simulink model "simple_kafka_consumer_producer_example"  (R2018a)
settings: Solver=FixedStepAuto  StartTime=0.0  StopTime=inf  RelTol=1e-3
libraries: simulink x5, sl_kafka_lib x4
settings Model: EnablePacing=on  Creator=asolland  LastModifiedBy=asolland
settings OptimizationCC: DefaultParameterBehavior=Inlined  EnhancedBackFolding=on  PassReuseOutputArgsAs=Individual arguments  OptimizeBlockOrder=speed  DifferentSizesBufferReuse=on  OptimizationCustomize=off
settings DebuggingCC: ParameterTunabilityLossMsg=error
settings HardwareCC: ProdBitPerLong=64  ProdLongLongMode=on  ProdHWDeviceType=Intel->x86-64 (Linux 64)
settings SFSimCC: SimUseLocalCustomCode=on  MATLABDynamicMemAlloc=off
settings RTWCC: Description=Kafka Target  SystemTargetFile=kafkatarget.tlc  TemplateMakefile=ert_default_tmf  GenerateReport=on  RetainRTWFile=on  RTWUseLocalCustomCode=on  IncludeHyperlinkInReport=on  LaunchReport=on  GenerateTraceInfo=on  GenerateTraceReport=on  GenerateTraceReportSl=on  GenerateTraceReportSf=on  GenerateTraceReportEml=on
settings CodeAppCC: ForceParamTrailComments=on  IgnoreCustomStorageClasses=off  OperatorAnnotations=on  SimulinkDataObjDesc=on  SFDataObjDesc=on  InsertBlockDesc=on
settings STFCustomTargetCC: TargetLangStandard=C99 (ISO)  MultiwordLength=256  GenerateSampleERTMain=on  CombineOutputUpdateFcns=on  ERTCustomFileBanners=on  SupportContinuousTime=off  SupportNonInlinedSFcns=off  RemoveResetFunc=on  MATLABClassNameForMDSCustomization=Simulink.SoftwareTarget.ERTCustomization  GRTInterface=off  UseToolchainInfoCompliant=on  SystemTargetFile=kafkatarget.tlc
settings ERTTargetCC: TargetLangStandard=C99 (ISO)  GenerateSampleERTMain=on  ParMdlRefBuildCompliant=off  CompOptLevelCompliant=off  ConcurrentExecutionCompliant=off  ModelStepFunctionPrototypeControlCompliant=off  CPPClassGenCompliant=off  InlinedParameterPlacement=NonHierarchical  ERTCustomFileTemplate=kafkatarget_process.tlc

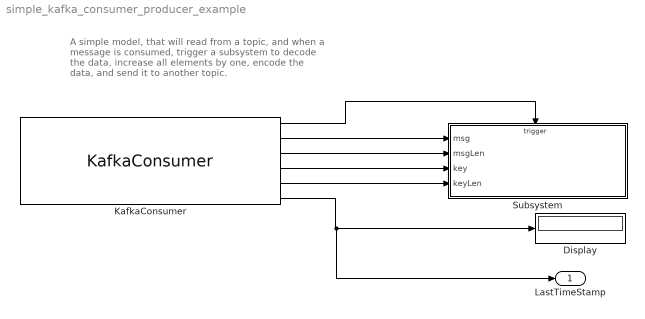
== system simple_kafka_consumer_producer_example ==
  note: A simple model, that will read from a topic, and
      | when a message is consumed, trigger a subsystem
      | to decode the data, increase all elements by one,
      | encode the data, and send it to another topic.
  Display : Display
  KafkaConsumer : sl_kafka_lib/KafkaConsumer  sfpBrokers='localhost:9092'  sfpTopic='sltopic'  sfpGroup='abc'  sfpMsgLen=200  sfpKeyLen=32  sfpOutputTimestamp=on  sfpTS=1e-3  sfpConf=|  sfpTopicConf=compression.level=-1
      | client.id=sl_kafka_consumer
      | message.copy.max.bytes=65535
      settings: SourceProductName=Kafka Library
  Subsystem : Subsystem
  LastTimeStamp : Outport  VectorParamsAs1DForOutWhenUnconnected=off
  wires:
  KafkaConsumer/2 -> Subsystem/1(msg)
  KafkaConsumer/3 -> Subsystem/2(msgLen)
  KafkaConsumer/4 -> Subsystem/3(key)
  KafkaConsumer/5 -> Subsystem/4(keyLen)
  KafkaConsumer/1 -> Subsystem/Trigger
  KafkaConsumer/6 -> LastTimeStamp/1, Display/1

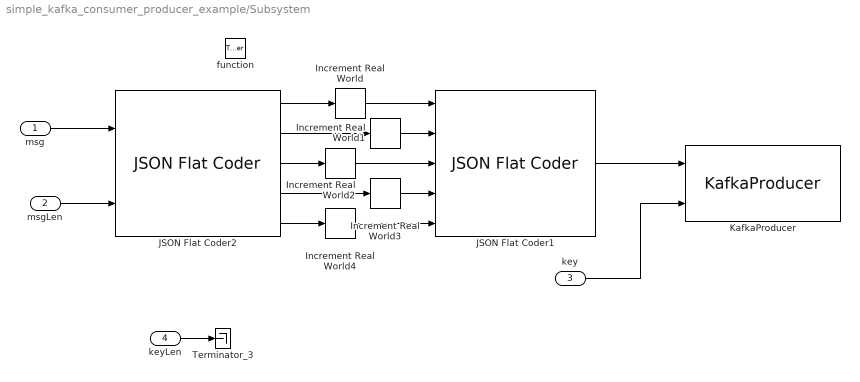
== system simple_kafka_consumer_producer_example/Subsystem ==
  msg : Inport
  msgLen : Inport  Port=2
  key : Inport  Port=3
  keyLen : Inport  Port=4
  function : TriggerPort  TriggerType=function-call  VariantControl=Variant
  Increment Real World{,1..4} (5 alike) : simulink/Additional Math & Discrete/Additional Math: Increment - Decrement/Increment Real World
      settings: SourceProductName=Simulink  SourceProductBaseCode=SL
  JSON Flat Coder1 : sl_kafka_lib/JSON Flat Coder  sfpDirection=Encode  sfpLength=200  sfpFields={'TS', 'M', 'Flow', 'Pressure', 'Current'}  sfpOutLength=off  sfpInLength=on
      settings: SourceProductName=Kafka Library
  JSON Flat Coder2 : sl_kafka_lib/JSON Flat Coder  sfpDirection=Decode  sfpLength=200  sfpFields={'TS', 'M', 'Flow', 'Pressure', 'Current'}  sfpOutLength=on  sfpInLength=on
      settings: SourceProductName=Kafka Library
  KafkaProducer : sl_kafka_lib/KafkaProducer  sfpBrokers='localhost:9092'  sfpTopic='sltopic2'  sfpKeyAsInput=on  sfpKeyAsInputLen=32  sfpKey='key1'  sfpMsgLen=200  sfpTS=-1  sfpConf=|  sfpTopicConf=compression.level=-1
      | client.id=sl_kafka_producer
      | message.copy.max.bytes=65535
      settings: SourceProductName=Kafka Library
  Terminator_3 : Terminator
  wires:
  msg/1 -> JSON Flat Coder2/1
  JSON Flat Coder2/1 -> Increment Real World/1
  JSON Flat Coder2/2 -> Increment Real World1/1
  JSON Flat Coder2/4 -> Increment Real World3/1
  JSON Flat Coder2/3 -> Increment Real World2/1
  JSON Flat Coder2/5 -> Increment Real World4/1
  msgLen/1 -> JSON Flat Coder2/2
  key/1 -> KafkaProducer/2
  keyLen/1 -> Terminator_3/1
  JSON Flat Coder1/1 -> KafkaProducer/1
  Increment Real World/1 -> JSON Flat Coder1/1
  Increment Real World1/1 -> JSON Flat Coder1/2
  Increment Real World2/1 -> JSON Flat Coder1/3
  Increment Real World3/1 -> JSON Flat Coder1/4
  Increment Real World4/1 -> JSON Flat Coder1/5
